simulink model "motor"  (R2022b)
settings: Solver=VariableStepAuto  StartTime=0.0  StopTime=50  RelTol=1e-3
libraries: spsDCMachineLib x1, spsACVoltageSourceLib x1, spsThyristorLib x1, spsVoltageMeasurementLib x1, spspowerguiLib x1
settings Model: Creator=user  LastModifiedBy=user
settings SolverCC: ZeroCrossAlgorithm=Adaptive
settings DebuggingCC: IgnoredZcDiagnostic=none

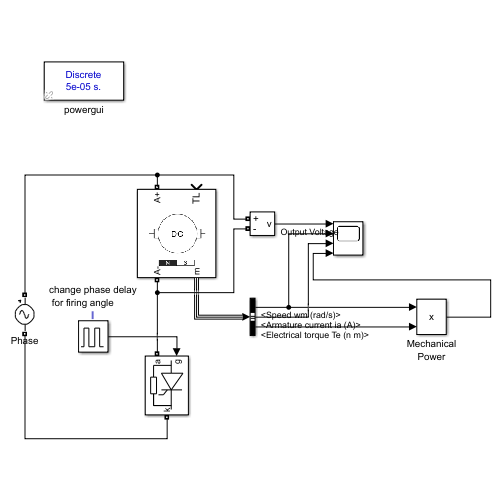
[thumbnail: Simulink's stored preview of the top-level diagram]
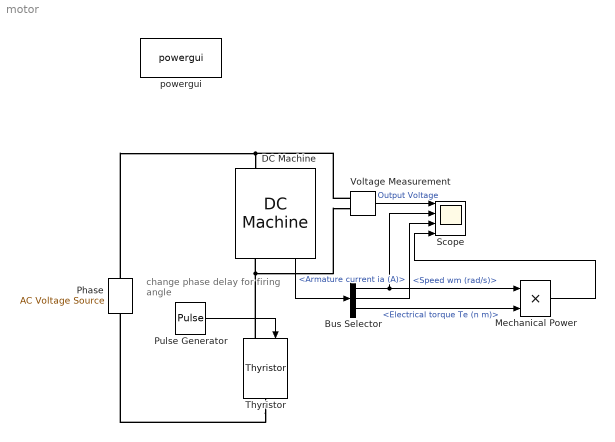
== system motor ==
  note: change phase delay
      |  for firing angle
  Bus Selector : BusSelector  OutputSignals=Speed wm (rad/s),Armature current ia (A),Electrical torque Te (n m)
  DC Machine : spsDCMachineLib/DC Machine  PresetModel=No  MechanicalLoad=Torque TL  FieldType=Permanent magnet  ShowDetailedParameters=on  MeasurementBus=off  RLa="[ 0.8  0.0125]"  RLf="[ 210  23]"  Laf=1.8  MachineConstant=Back-emf constant (V/rpm)  Ke=220/1500  Kt=1.8  J=1  Bm=0.12  Tf=1.59  w0=0  Ifinit=1  TsPowergui=0  TsBlock=-1
  Mechanical Power : Product
  Phase : spsACVoltageSourceLib/AC Voltage Source  Amplitude=400  Phase=0  Frequency=50  SampleTime=0  Measurements=None  BusType=swing  Pref=10e3  Qref=0  Qmin=-inf  Qmax=+inf
  Pulse Generator : DiscretePulseGenerator  PulseType=Time based  Period=20e-3  PulseWidth=5  PhaseDelay=7e-3
  Scope : Scope  NumInputPorts=4
  Thyristor : spsThyristorLib/Thyristor  Ron=0.001  Lon=0  Vf=0.8  IC=0  Rs=500  Cs=250e-9  Measurements=off
  Voltage Measurement : spsVoltageMeasurementLib/Voltage Measurement  PhasorSimulation=off  OutputType=Complex  PSBequivalent=0
  powergui : spspowerguiLib/powergui  Priority=1  SimulationMode=Discrete  SampleTime=50e-6  frequency=60  Iterations=50  frequencyindice=50  Pbase=100e6  ErrMax=1e-4  UnitsV=kV  UnitsW=MW  buscounter=0  FunctionMessages=off  echomessages=off  EnableUseOfTLC=off  CurrentSourceSwitches=off  DisableSnubberDevices=off  DisableRonSwitches=off  DisableVfSwitches=off  DisplayEquations=off  AutomaticDiscreteSolvers=off  SolverType=Tustin/Backward Euler (TBE)  Interpol=off  ExternalGateDelay=off  methode=off  Ts=100  x0status=blocks  SPID=on  SwTol=0  HookPort=off  NonlinearTolerance=1e-4  nMaxIteration=100  ContinueOnMaxIteration=off  RestoreLinks=warning  ResistiveCurrentMeasurement=off  Frange=[0:2:500]  Ylog=off  Xlog=on  ShowGrid=off  save=off  variable=ZData  structure=0  ZoomFFT=off  StartTime=0.0  cycles=1  DisplayStyle=1  fundamental=60  FreqAxis=off  MaxFrequency=1000  frequencyindicesteady=1  RmsSteady=1  display=off
  wires:
  DC Machine/1 -> Bus Selector/1
  Bus Selector/1 -> Mechanical Power/1, Scope/2  "<Speed wm (rad/s)>"
  Voltage Measurement/1 -> Scope/1  "Output Voltage"
  Pulse Generator/1 -> Thyristor/1
  Bus Selector/2 -> Scope/3  "<Armature current ia (A)>"
  Bus Selector/3 -> Mechanical Power/2  "<Electrical torque Te (n m)>"
  Mechanical Power/1 -> Scope/4
  connections:
  Thyristor/LConn1 -- Voltage Measurement/LConn2 -- DC Machine/RConn1
  Thyristor/RConn1 -- Phase/LConn1
  Phase/RConn1 -- Voltage Measurement/LConn1 -- DC Machine/LConn1
